simulink model "P1"  (R2021b)
settings: Solver=ode1  StartTime=0.0  StopTime=10.0  FixedStep=0.1  RelTol=1e-3
values from neighbouring files (symbols this model uses):
  D = 0.1*eye(3)    [p2v1.m]
libraries: sharedutil x1
settings Model: Creator=dedo  LastModifiedBy=dedo
settings DataIOCC: ReturnWorkspaceOutputs=off

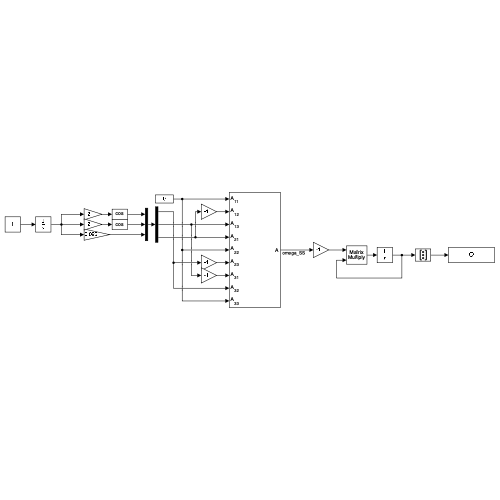
[thumbnail: Simulink's stored preview of the top-level diagram]
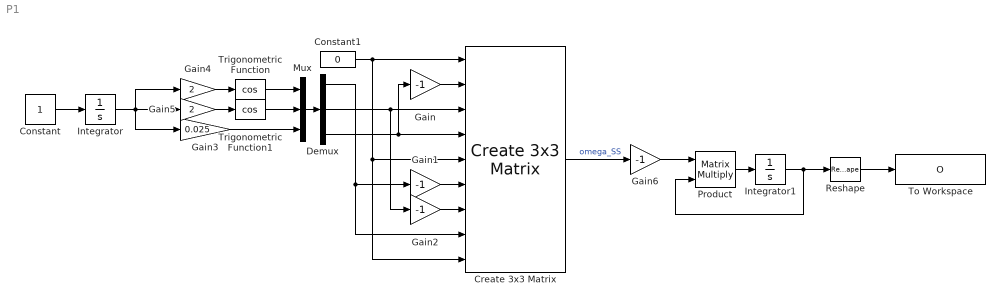
== system P1 ==
  Constant : Constant
  Constant1 : Constant  Value=0
  Create 3x3 Matrix : sharedutil/Create 3x3 Matrix  aMode=aMode
      settings: SourceProductBaseCode=AE,PW,DR,MT,UV,VE
  Demux : Demux  Outputs=3
  Gain{,1..2,6} (4 alike) : Gain  Gain=-1
  Gain3 : Gain  Gain=0.025
  Gain4 : Gain  Gain=2
  Gain5 : Gain  Gain=2
  Integrator : Integrator
  Integrator1 : Integrator  InitialCondition=eye(3)
  Mux : Mux  Inputs=3
  Product : Product  Multiplication=Matrix(*)
  Reshape : Reshape  OutputDimensionality=Column vector (2-D)
  To Workspace : ToWorkspace  VariableName=O  SampleTime=-1
  Trigonometric Function : Trigonometry  Operator=cos
  Trigonometric Function1 : Trigonometry  Operator=cos
  wires:
  Constant1/1 -> Create 3x3 Matrix/1, Create 3x3 Matrix/5, Create 3x3 Matrix/9
  Gain/1 -> Create 3x3 Matrix/2
  Gain1/1 -> Create 3x3 Matrix/6
  Gain2/1 -> Create 3x3 Matrix/7
  Demux/1 -> Gain1/1, Create 3x3 Matrix/8
  Demux/3 -> Create 3x3 Matrix/4, Gain/1
  Demux/2 -> Create 3x3 Matrix/3, Gain2/1
  Mux/1 -> Demux/1
  Trigonometric Function/1 -> Mux/1
  Trigonometric Function1/1 -> Mux/2
  Gain3/1 -> Mux/3
  Constant/1 -> Integrator/1
  Integrator/1 -> Gain3/1, Gain4/1, Gain5/1
  Create 3x3 Matrix/1 -> Gain6/1  "omega_SS"
  Product/1 -> Integrator1/1
  Reshape/1 -> To Workspace/1
  Integrator1/1 -> Reshape/1, Product/2
  Gain4/1 -> Trigonometric Function/1
  Gain5/1 -> Trigonometric Function1/1
  Gain6/1 -> Product/1
